simulink model "EX_2_4"  (R2024b)
settings: Solver=FixedStepAuto  StartTime=0.0  StopTime=total_time  FixedStep=Ts  RelTol=1e-3
undefined symbols (not defined in the file): q, Ts
settings Model: Creator=alber  LastModifiedBy=Enrico
settings RTWCC: GPUComputeCapability=3.5

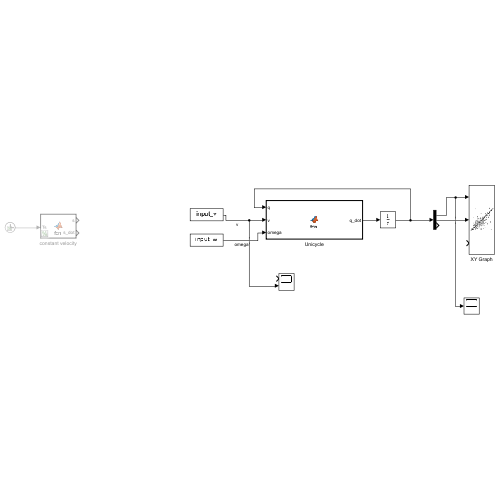
[thumbnail: Simulink's stored preview of the top-level diagram]
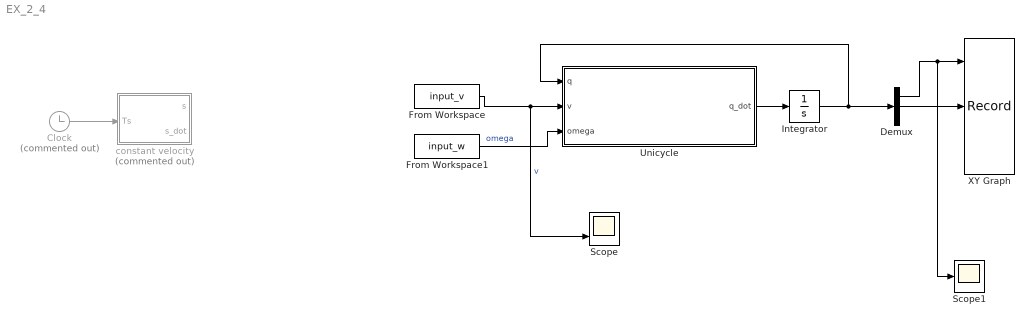
== system EX_2_4 ==
  Clock : Clock  Commented=on
  Demux : Demux  Outputs=3
  From Workspace : FromWorkspace  VariableName=input_v  SampleTime=Ts
  From Workspace1 : FromWorkspace  VariableName=input_w  SampleTime=Ts
  Integrator : Integrator  InitialCondition=[q(1,1);q(2,1);q(3,1)]
  Scope : Scope  NumInputPorts=2
  Scope1 : Scope
  Unicycle : MATLAB Function  TreatAsAtomicUnit=on
  XY Graph : Record  FileSettingsInternal="{\"entries\":[{\"content\":{\"excelSettings\":{\"content\":{},\"type\":\"Streamout.ExcelSettings\"}},\"type\":\"Streamout.FileSettingStorage\",\"uuid\":\"\"}],\"packageUris\":[\"http:\\/\\/schema.mathworks.com\\/mf0\\/streamout_blocks\\/R2020a\"],\"version\":\"1.0\"}"  Layout=[1 1]  SignalsInternal="{\"entries\":[{\"content\":{\"signals\":[{\"content\":{\"blockPath\":[],\"dimensions\":[1,1],\"domain\":\"\",\"lineColor\":\"#7e2f8e\",\"lineWidth\":2,\"plots\":[ 1 ],\"port\":1,\"sid\":[\"\"],\"signalID\":1,\"signalName\":\"Demux:1\"},\"type\":\"RecordBlkView.Signal\",\"uuid\":\"\"},{\"content\":{\"blockPath\":[],\"dimensions\":[1,1],\"domain\":\"\",\"lineColor\":\"#77ac30\",\"lineWidth\":2,\"plots\":[ 1 ],\"port\":2,\"sid\":[\"\"],\"signalID\":2,\"signalName\":\"Demux:2\"},\"type\":\"RecordBlkView.Signal\",\"uuid\":\"\"},{\"content\":{\"blockPath\":[],\"dimensions\":[1],\"domain\":\"\",\"lineColor\":\"#4dbeee\",\"lineWidth\":2,\"port\":3,\"sid\":[\"\"],\"signalID\":3},\"type\":\"RecordBlkView.Signal\",\"uuid\":\"\"}]},\"type\":\"RecordBlkView.InputSignals\",\"uuid\":\"\"}],\"packageUris\":[\"http:\\/\\/schema.mathworks.com\\/mf0\\/streamout_blocks\\/R2020a\"],\"version\":\"1.0\"}"  VisualizationBindings="{\"xyplotplugin\":{\"info\":[{\"series\":[{\"bindingParametersList\":[{\"parameter\":\"X-Axis\",\"signalID\":1,\"signalName\":\"Demux:1\"},{\"parameter\":\"X-Axis\",\"signalID\":1,\"signalName\":\"Demux:1\"},{\"parameter\":\"Y-Axis\",\"signalID\":2,\"signalName\":\"Demux:2\"}],\"seriesID\":0}],\"subplotID\":1}]}}"  CompatibilityTag=XY
  constant velocity : MATLAB Function  Commented=on  TreatAsAtomicUnit=on
  wires:
  Unicycle/1(q_dot) -> Integrator/1
  Integrator/1 -> Unicycle/1(q), Demux/1
  Demux/1 -> Scope1/1, XY Graph/1
  Demux/2 -> XY Graph/2
  Clock/1 -> constant velocity/1(Ts)
  From Workspace1/1 -> Unicycle/3(omega)  "omega"
  From Workspace/1 -> Scope/2, Unicycle/2(v)  "v"

== matlab function EX_2_4/Unicycle ==
  data: q_dot output; q input; v input; omega input
function q_dot = fcn(q, v, omega)
q_dot = [cos(q(3))*v; sin(q(3))*v; omega];

== matlab function EX_2_4/constant velocity ==
  data: Ts input; s output; s_dot output; total_time parameter
function [s, s_dot] = fcn(Ts,total_time)

s_dot = 1/total_time;
s= Ts/total_time;
